simulink model "dspsdadc"  (R2014a)
settings: Solver=ode5  SolverMode=SingleTasking  StartTime=0.0  StopTime=inf  MaxStep=1/512000  RelTol=1e-3  AbsTol=1e-6
libraries: dspmlti4 x3, dsparch4 x2, dspmisc x1
settings Model: PauseTimes=0.025  ExtModeTrigMode=oneshot  ExtModeArmWhenConnect=off  ExtModeAutoUpdateStatusClock=off  Creator=The MathWorks Inc.  LastModifiedBy=of-1
settings DataIOCC: LimitDataPoints=off  SignalLoggingSaveFormat=ModelDataLogs  SaveOutput=off  SaveTime=off  SignalLoggingName=logsOut
settings OptimizationCC: BlockReduction=off  BooleanDataType=off  ExpressionDepthLimit=2147483647  RollThreshold=2  InitFltsAndDblsToZero=on  EfficientMapNaN2IntZero=off
settings DebuggingCC: SaveWithParameterizedLinksMsg=none  UnderspecifiedInitializationDetection=Classic  SignalResolutionControl=TryResolveAllWithWarning  SolverPrmCheckMsg=none  MultiTaskDSMMsg=warning  MultiTaskCondExecSysMsg=none  IntegerOverflowMsg=none  FcnCallInpInsideContextMsg=UseLocalSettings  StateNameClashWarn=warning
settings HardwareCC: TargetUnknown=on
settings RTWCC: IncludeERTFirstTime=on
settings GRTTargetCC: TargetFcnLib=ansi_tfl_tmw.mat  CombineOutputUpdateFcns=off  GRTInterface=on

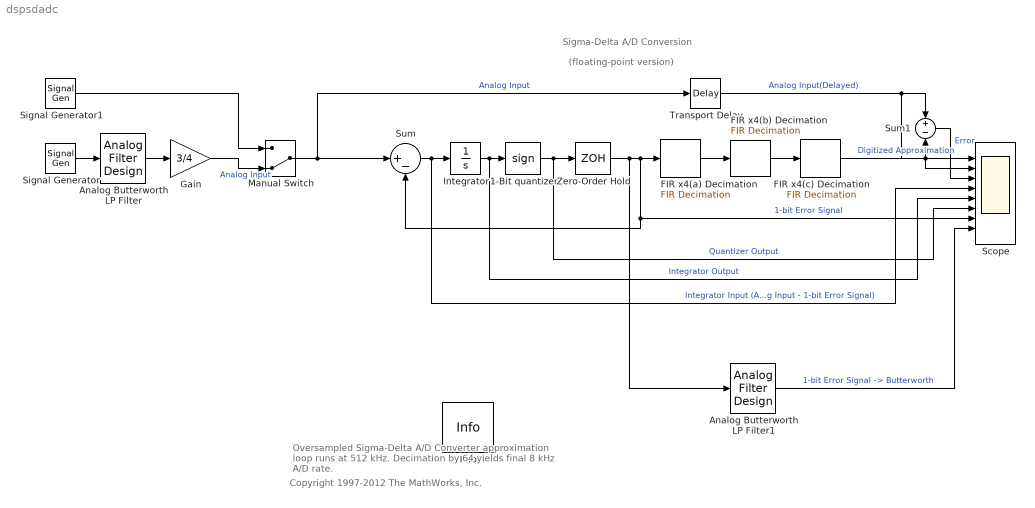
== system dspsdadc ==
  note: Oversampled Sigma-Delta A/D Converter
      | approximation loop runs at 512 kHz.
      | Decimation by 64 yields final 8 kHz A/D rate.
  note: Copyright 1997-2012 The MathWorks, Inc.
  note: Sigma-Delta A/D Conversion
  note: (floating-point version)
  1-Bit quantizer : Signum
  Analog Butterworth LP Filter : dsparch4/Analog Filter Design  method=Butterworth  filttype=Lowpass  N=5  Wlo=2*pi*200  Whi=80  Rp=2  Rs=40
  Analog Butterworth LP Filter1 : dsparch4/Analog Filter Design  method=Butterworth  filttype=Lowpass  N=5  Wlo=2*pi*400  Whi=80  Rp=2  Rs=40
  FIR x4(a) Decimation : dspmlti4/FIR Decimation  h=fir1(31,0.15)  D=4  filtStruct=Direct form  framing=Maintain input frame size  inputOffset=0  outputBufInitCond=0  firstCoeffDataTypeStr=Inherit: Same word length as input  firstCoeffLastDataTypeStr=Inherit: Same word length as input  firstCoeffMin=[]  firstCoeffMax=[]  outputMin=[]  outputMax=[]  accumDataTypeStr=Inherit: Same as product output  accumLastDataTypeStr=Inherit: Same as product output  roundingMode=Floor  overflowMode=off  FilterSource=Specify via dialog  FilterObject=Hm_firdecim
  FIR x4(b) Decimation : dspmlti4/FIR Decimation  h=fir1(31,0.15)  D=4  filtStruct=Direct form  framing=Maintain input frame size  inputOffset=0  outputBufInitCond=0  firstCoeffDataTypeStr=Inherit: Same word length as input  firstCoeffLastDataTypeStr=Inherit: Same word length as input  firstCoeffMin=[]  firstCoeffMax=[]  outputMin=[]  outputMax=[]  accumDataTypeStr=Inherit: Same as product output  accumLastDataTypeStr=Inherit: Same as product output  roundingMode=Floor  overflowMode=off  FilterSource=Specify via dialog  FilterObject=Hm_firdecim
  FIR x4(c) Decimation : dspmlti4/FIR Decimation  h=fir1(31,0.15)  D=4  filtStruct=Direct form  framing=Maintain input frame size  inputOffset=0  outputBufInitCond=0  firstCoeffDataTypeStr=Inherit: Same word length as input  firstCoeffLastDataTypeStr=Inherit: Same word length as input  firstCoeffMin=[]  firstCoeffMax=[]  outputMin=[]  outputMax=[]  accumDataTypeStr=Inherit: Same as product output  accumLastDataTypeStr=Inherit: Same as product output  roundingMode=Floor  overflowMode=off  FilterSource=Specify via dialog  FilterObject=Hm_firdecim
  Gain : Gain  Gain=3/4  SaturateOnIntegerOverflow=on  OutDataTypeStr=Inherit: Same as input  ParamDataTypeStr=Inherit: Same as input
  Info : dspmisc/Info  SystemSampleTime=-1
  Integrator : Integrator
  Manual Switch : ManualSwitch  CurrentSetting=0
  Scope : Scope  NumInputPorts=8
      settings: TimeRange=0.025  YMin=-1~-1.25~-1~-2~-4e-06~-1.3~-1.3~-1.3  YMax=1~1.25~1~2~4e-06~1.3~1.3~1.3  MaxDataPoints=15000  SampleTime=1
  Signal Generator : SignalGenerator  WaveForm=square  Frequency=80
  Signal Generator1 : SignalGenerator  WaveForm=square  Frequency=80
  Sum : Sum  Inputs=|+-  SaturateOnIntegerOverflow=on  InputSameDT=on  OutDataTypeStr=Inherit: Same as first input
  Sum1 : Sum  Inputs=+-  SaturateOnIntegerOverflow=on  InputSameDT=on  OutDataTypeStr=Inherit: Same as first input
  Transport Delay : TransportDelay  DelayTime=336/512000
  Zero-Order Hold : ZeroOrderHold  SampleTime=1/512000
  wires:
  Zero-Order Hold/1 -> Analog Butterworth LP Filter1/1, FIR x4(a) Decimation/1, Scope/7, Sum/2  "1-bit Error Signal"
  FIR x4(c) Decimation/1 -> Scope/2, Sum1/2  "Digitized Approximation"
  Analog Butterworth LP Filter/1 -> Gain/1
  Signal Generator/1 -> Analog Butterworth LP Filter/1
  FIR x4(a) Decimation/1 -> FIR x4(b) Decimation/1
  FIR x4(b) Decimation/1 -> FIR x4(c) Decimation/1
  Sum1/1 -> Scope/3  "Error"
  Transport Delay/1 -> Sum1/1, Scope/1  "Analog Input(Delayed)"
  1-Bit quantizer/1 -> Scope/6, Zero-Order Hold/1  "Quantizer Output"
  Sum/1 -> Scope/4, Integrator/1  "Integrator Input (Analog Input - 1-bit Error Signal)"
  Integrator/1 -> Scope/5, 1-Bit quantizer/1  "Integrator Output"
  Gain/1 -> Manual Switch/2  "Analog Input"
  Manual Switch/1 -> Transport Delay/1, Sum/1  "Analog Input"
  Analog Butterworth LP Filter1/1 -> Scope/8  "1-bit Error Signal -> Butterworth"
  Signal Generator1/1 -> Manual Switch/1
